simulink model "TestCase1_Modified"  (R2014a)
settings: Solver=FixedStepAuto  StartTime=0.0  StopTime=10.0  RelTol=1e-3
model workspace: external: MAT-File TestCase1.mat (data not in the file)
libraries: libAsserts x5
settings Model: Creator=Josef  LastModifiedBy=swami
settings DataIOCC: SaveFormat=Dataset
settings OptimizationCC: SimCompilerOptimization=off
settings DebuggingCC: MergeDetectMultiDrivingBlocksExec=error  SolverPrmCheckMsg=none  FrameProcessingCompatibilityMsg=error  AllowSymbolicDim=off
settings HardwareCC: ProdBitPerPointer=64  ProdLargestAtomicFloat=Float  ProdIntDivRoundTo=Zero  ProdEndianess=LittleEndian  ProdWordSize=64  ProdHWDeviceType=Intel->x86-64 (Windows64)
settings RTWCC: RTWCompilerOptimization=off
settings GRTTargetCC: GeneratePreprocessorConditionals=Use local settings
settings ConfigComp: CovMetricSettings=dw  CovHtmlReporting=on  CovSaveCumulativeToWorkspaceVar=on  CovSaveSingleToWorkspaceVar=on  CovExternalEMLEnable=off

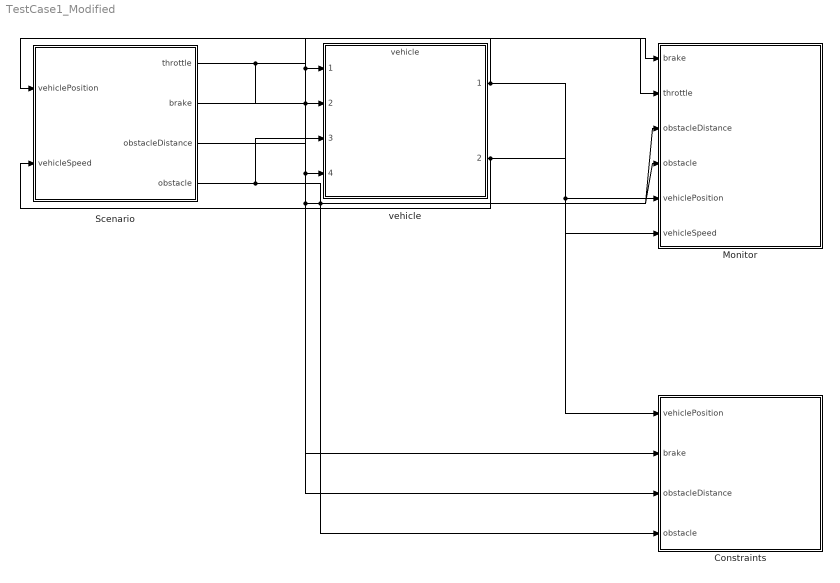
== system TestCase1_Modified ==
  Constraints : Subsystem
  Monitor : Subsystem
  Scenario : Subsystem
  vehicle : ModelReference  ModelNameDialog=vehicle  SimulationMode=Normal  ModelReferenceVersion=1.16  CopyOfModelName=vehicle  DefaultDataLogging=on
  wires:
  Scenario/1(throttle) -> vehicle/2, Monitor/2(throttle)
  Scenario/2(brake) -> vehicle/1, Monitor/1(brake), Constraints/2(brake)
  Scenario/4(obstacle) -> Monitor/4(obstacle), Constraints/4(obstacle), vehicle/3
  Scenario/3(obstacleDistance) -> Monitor/3(obstacleDistance), Constraints/3(obstacleDistance), vehicle/4
  vehicle/2 -> Scenario/2(vehicleSpeed), Monitor/6(vehicleSpeed)
  vehicle/1 -> Monitor/5(vehiclePosition), Constraints/1(vehiclePosition), Scenario/1(vehiclePosition)

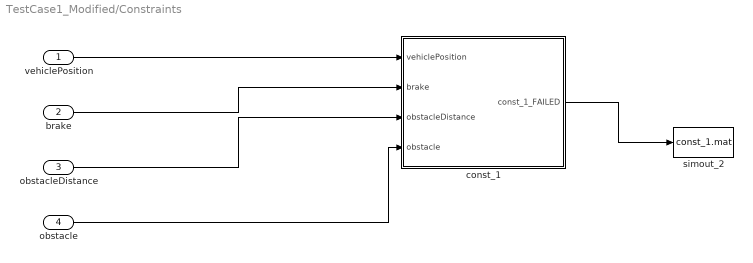
== system TestCase1_Modified/Constraints ==
  vehiclePosition : Inport
  brake : Inport  Port=2
  obstacleDistance : Inport  Port=3
  obstacle : Inport  Port=4
  const_1 : Subsystem
  simout_2 : ToFile  Filename=const_1.mat  MatrixName=const_1  SaveFormat=Timeseries
  wires:
  vehiclePosition/1 -> const_1/1(vehiclePosition)
  obstacleDistance/1 -> const_1/3(obstacleDistance)
  obstacle/1 -> const_1/4(obstacle)
  const_1/1(const_1_FAILED) -> simout_2/1
  brake/1 -> const_1/2(brake)

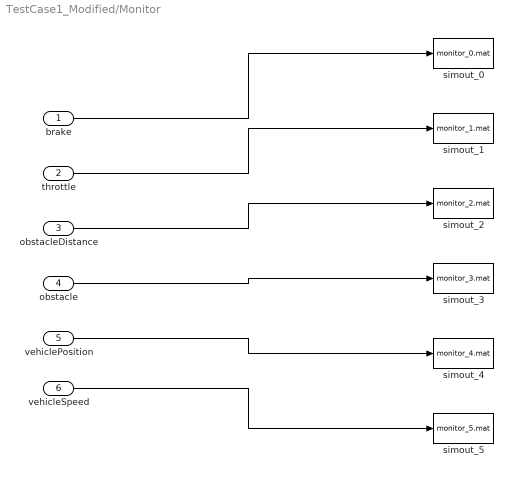
== system TestCase1_Modified/Monitor ==
  brake : Inport
  throttle : Inport  Port=2
  obstacleDistance : Inport  Port=3
  obstacle : Inport  Port=4
  vehiclePosition : Inport  Port=5
  vehicleSpeed : Inport  Port=6
  simout_0 : ToFile  Filename=monitor_0.mat  MatrixName=brake  SaveFormat=Timeseries
  simout_1 : ToFile  Filename=monitor_1.mat  MatrixName=throttle  SaveFormat=Timeseries
  simout_2 : ToFile  Filename=monitor_2.mat  MatrixName=obstacleDistance  SaveFormat=Timeseries
  simout_3 : ToFile  Filename=monitor_3.mat  MatrixName=obstacle  SaveFormat=Timeseries
  simout_4 : ToFile  Filename=monitor_4.mat  MatrixName=vehiclePosition  SaveFormat=Timeseries
  simout_5 : ToFile  Filename=monitor_5.mat  MatrixName=vehicleSpeed  SaveFormat=Timeseries
  wires:
  brake/1 -> simout_0/1
  throttle/1 -> simout_1/1
  obstacleDistance/1 -> simout_2/1
  obstacle/1 -> simout_3/1
  vehiclePosition/1 -> simout_4/1
  vehicleSpeed/1 -> simout_5/1

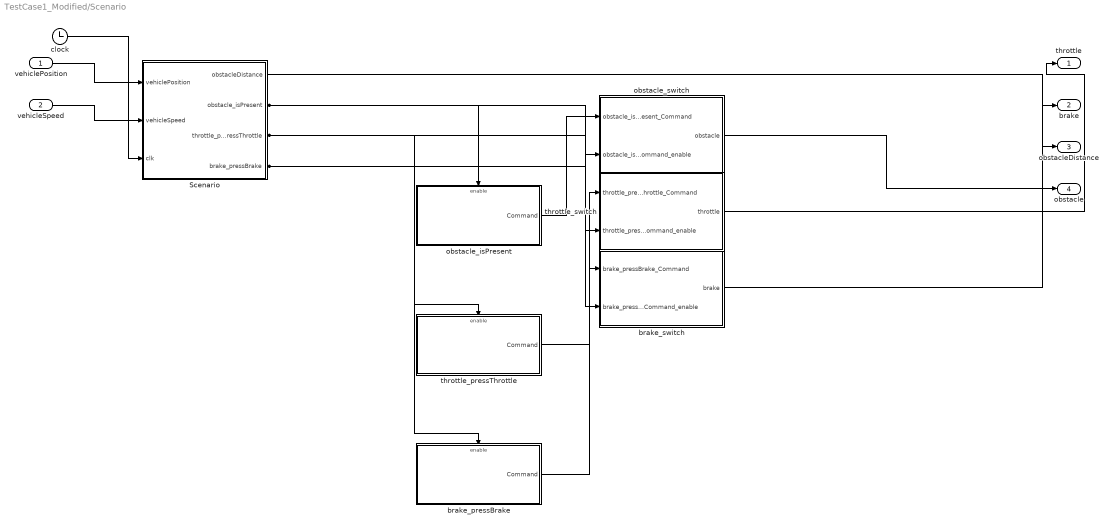
== system TestCase1_Modified/Scenario ==
  vehiclePosition : Inport
  vehicleSpeed : Inport  Port=2
  Scenario : Stateflow chart  TreatAsAtomicUnit=on
  brake_pressBrake : Subsystem
  brake_switch : Subsystem
  clock : Clock
  obstacle_isPresent : Subsystem
  obstacle_switch : Subsystem
  throttle_pressThrottle : Subsystem
  throttle_switch : Subsystem
  throttle : Outport
  brake : Outport  Port=2
  obstacleDistance : Outport  Port=3
  obstacle : Outport  Port=4
  wires:
  obstacle_switch/1(obstacle) -> obstacle/1
  throttle_switch/1(throttle) -> throttle/1
  brake_switch/1(brake) -> brake/1
  obstacle_isPresent/1(Command) -> obstacle_switch/1(obstacle_isPresent_Command)
  Scenario/2(obstacle_isPresent) -> obstacle_switch/2(obstacle_isPresent_Command_enable), obstacle_isPresent/Enable
  throttle_pressThrottle/1(Command) -> throttle_switch/1(throttle_pressThrottle_Command)
  Scenario/3(throttle_pressThrottle) -> throttle_switch/2(throttle_pressThrottle_Command_enable), throttle_pressThrottle/Enable
  brake_pressBrake/1(Command) -> brake_switch/1(brake_pressBrake_Command)
  Scenario/4(brake_pressBrake) -> brake_switch/2(brake_pressBrake_Command_enable), brake_pressBrake/Enable
  Scenario/1(obstacleDistance) -> obstacleDistance/1
  vehicleSpeed/1 -> Scenario/2(vehicleSpeed)
  vehiclePosition/1 -> Scenario/1(vehiclePosition)
  clock/1 -> Scenario/3(clk)

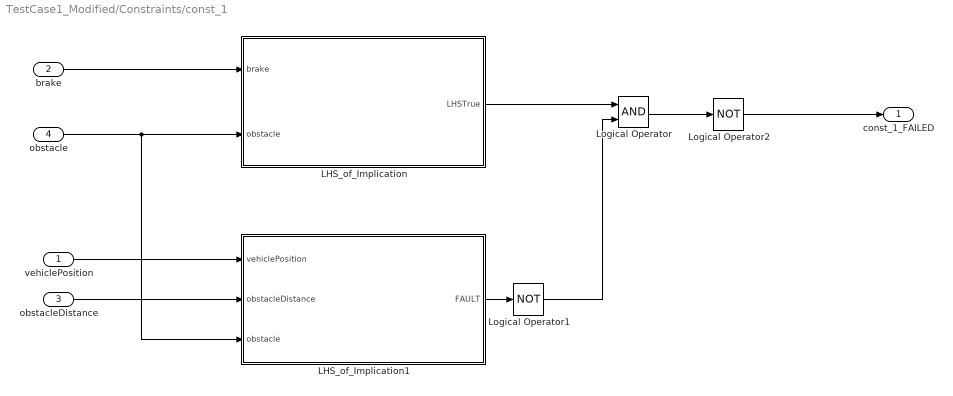
== system TestCase1_Modified/Constraints/const_1 ==
  vehiclePosition : Inport
  brake : Inport  Port=2
  obstacleDistance : Inport  Port=3
  obstacle : Inport  Port=4
  LHS_of_Implication : Subsystem
  LHS_of_Implication1 : Subsystem
  Logical Operator : Logic  AllPortsSameDT=off  OutDataTypeStr=boolean
  Logical Operator1 : Logic  Operator=NOT  AllPortsSameDT=off  OutDataTypeStr=boolean
  Logical Operator2 : Logic  Operator=NOT  AllPortsSameDT=off  OutDataTypeStr=boolean
  const_1_FAILED : Outport
  wires:
  brake/1 -> LHS_of_Implication/1(brake)
  obstacleDistance/1 -> LHS_of_Implication1/2(obstacleDistance)
  obstacle/1 -> LHS_of_Implication1/3(obstacle), LHS_of_Implication/2(obstacle)
  LHS_of_Implication1/1(FAULT) -> Logical Operator1/1
  LHS_of_Implication/1(LHSTrue) -> Logical Operator/1
  Logical Operator1/1 -> Logical Operator/2
  vehiclePosition/1 -> LHS_of_Implication1/1(vehiclePosition)
  Logical Operator/1 -> Logical Operator2/1
  Logical Operator2/1 -> const_1_FAILED/1

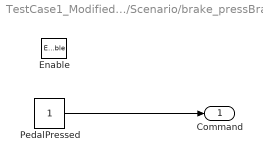
== system TestCase1_Modified/Scenario/brake_pressBrake ==
  Enable : EnablePort
  PedalPressed : Constant
  Command : Outport  OutputWhenDisabled=reset  InitialOutput=0
  wires:
  PedalPressed/1 -> Command/1

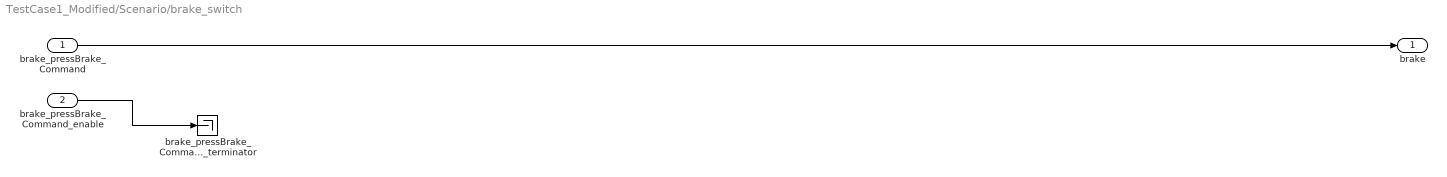
== system TestCase1_Modified/Scenario/brake_switch ==
  brake_pressBrake_Command : Inport
  brake_pressBrake_Command_enable : Inport  Port=2
  brake_pressBrake_Command_terminator : Terminator
  brake : Outport
  wires:
  brake_pressBrake_Command_enable/1 -> brake_pressBrake_Command_terminator/1
  brake_pressBrake_Command/1 -> brake/1

== system TestCase1_Modified/Scenario/obstacle_isPresent ==
  Enable : EnablePort
  PedalPressed : Constant
  Command : Outport  OutputWhenDisabled=reset  InitialOutput=0
  wires:
  PedalPressed/1 -> Command/1

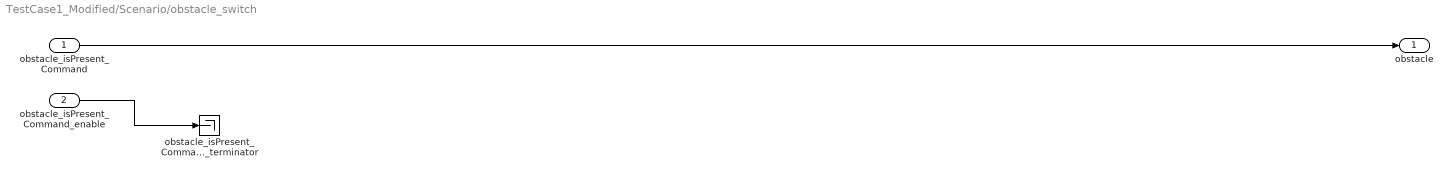
== system TestCase1_Modified/Scenario/obstacle_switch ==
  obstacle_isPresent_Command : Inport
  obstacle_isPresent_Command_enable : Inport  Port=2
  obstacle_isPresent_Command_terminator : Terminator
  obstacle : Outport
  wires:
  obstacle_isPresent_Command_enable/1 -> obstacle_isPresent_Command_terminator/1
  obstacle_isPresent_Command/1 -> obstacle/1

== system TestCase1_Modified/Scenario/throttle_pressThrottle ==
  Enable : EnablePort
  PedalPressed : Constant
  Command : Outport  OutputWhenDisabled=reset  InitialOutput=0
  wires:
  PedalPressed/1 -> Command/1

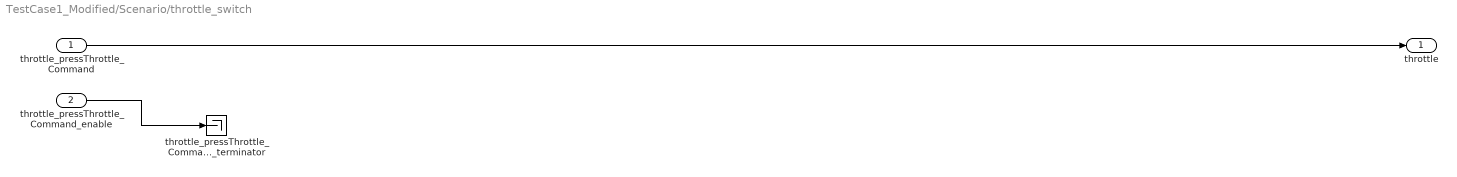
== system TestCase1_Modified/Scenario/throttle_switch ==
  throttle_pressThrottle_Command : Inport
  throttle_pressThrottle_Command_enable : Inport  Port=2
  throttle_pressThrottle_Command_terminator : Terminator
  throttle : Outport
  wires:
  throttle_pressThrottle_Command_enable/1 -> throttle_pressThrottle_Command_terminator/1
  throttle_pressThrottle_Command/1 -> throttle/1

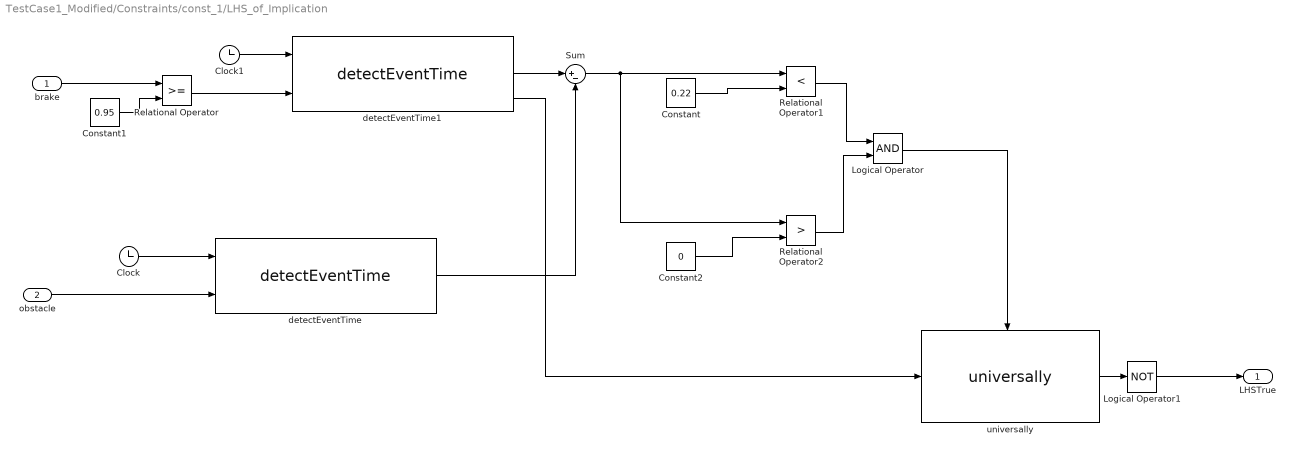
== system TestCase1_Modified/Constraints/const_1/LHS_of_Implication ==
  brake : Inport
  obstacle : Inport  Port=2
  Clock : Clock
  Clock1 : Clock
  Constant : Constant  Value=0.22
  Constant1 : Constant  Value=0.95
  Constant2 : Constant  Value=0
  Logical Operator : Logic  AllPortsSameDT=off  OutDataTypeStr=boolean
  Logical Operator1 : Logic  Operator=NOT  AllPortsSameDT=off  OutDataTypeStr=boolean
  Relational Operator : RelationalOperator  OutDataTypeStr=boolean
  Relational Operator1 : RelationalOperator  Operator=<  OutDataTypeStr=boolean
  Relational Operator2 : RelationalOperator  Operator=>  OutDataTypeStr=boolean
  Sum : Sum  Inputs=|+-
  detectEventTime : libAsserts/detectEventTime
  detectEventTime1 : libAsserts/detectEventTime
  universally : libAsserts/universally
  LHSTrue : Outport
  wires:
  detectEventTime1/2 -> Sum/1
  obstacle/1 -> detectEventTime/2
  universally/1 -> Logical Operator1/1
  Constant2/1 -> Relational Operator2/2
  Logical Operator1/1 -> LHSTrue/1
  Logical Operator/1 -> universally/Enable
  detectEventTime1/3 -> universally/1
  Sum/1 -> Relational Operator2/1, Relational Operator1/1
  Constant/1 -> Relational Operator1/2
  Relational Operator/1 -> detectEventTime1/2
  Clock1/1 -> detectEventTime1/1
  brake/1 -> Relational Operator/1
  Relational Operator1/1 -> Logical Operator/1
  detectEventTime/2 -> Sum/2
  Relational Operator2/1 -> Logical Operator/2
  Constant1/1 -> Relational Operator/2
  Clock/1 -> detectEventTime/1

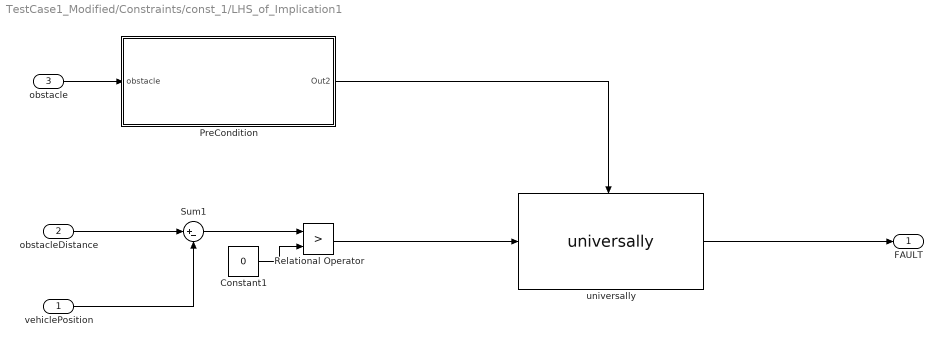
== system TestCase1_Modified/Constraints/const_1/LHS_of_Implication1 ==
  vehiclePosition : Inport
  obstacleDistance : Inport  Port=2
  obstacle : Inport  Port=3
  Constant1 : Constant  Value=0
  PreCondition : Subsystem
  Relational Operator : RelationalOperator  Operator=>  OutDataTypeStr=boolean
  Sum1 : Sum  Inputs=|+-
  universally : libAsserts/universally
  FAULT : Outport
  wires:
  Constant1/1 -> Relational Operator/2
  universally/1 -> FAULT/1
  obstacle/1 -> PreCondition/1(obstacle)
  obstacleDistance/1 -> Sum1/1
  vehiclePosition/1 -> Sum1/2
  Sum1/1 -> Relational Operator/1
  Relational Operator/1 -> universally/1
  PreCondition/1(Out2) -> universally/Enable

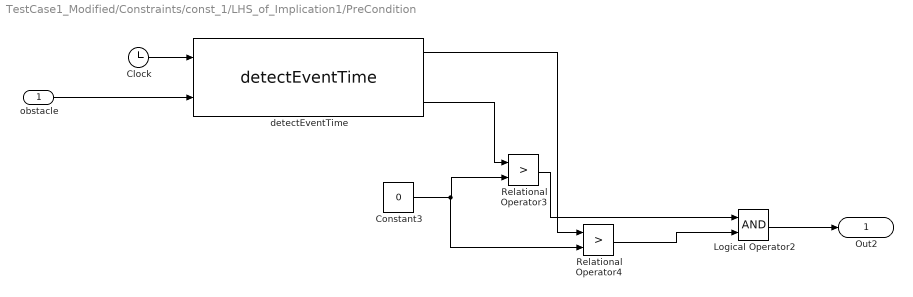
== system TestCase1_Modified/Constraints/const_1/LHS_of_Implication1/PreCondition ==
  obstacle : Inport
  Clock : Clock
  Constant3 : Constant  Value=0
  Logical Operator2 : Logic  AllPortsSameDT=off  OutDataTypeStr=boolean
  Relational Operator3 : RelationalOperator  Operator=>  OutDataTypeStr=boolean
  Relational Operator4 : RelationalOperator  Operator=>  OutDataTypeStr=boolean
  detectEventTime : libAsserts/detectEventTime
  Out2 : Outport
  wires:
  Clock/1 -> detectEventTime/1
  obstacle/1 -> detectEventTime/2
  Relational Operator3/1 -> Logical Operator2/1
  detectEventTime/1 -> Relational Operator4/1
  detectEventTime/3 -> Relational Operator3/1
  Constant3/1 -> Relational Operator4/2, Relational Operator3/2
  Logical Operator2/1 -> Out2/1
  Relational Operator4/1 -> Logical Operator2/2

== stateflow chart TestCase1_Modified/Scenario/Scenario ==
  state Act_Driver [parallel]
    settings: executionOrder=1
    state Act_Driver_Step1
      state Act_Driver_Step1_1
        entry: throttle_pressThrottle = 1;
      state Act_Driver_Step1_2
        entry: throttle_pressThrottle = 0;
      (default) -> Act_Driver_Step1_1
      Act_Driver_Step1_1 -> Act_Driver_Step1_2 : [vehicleSpeed >= 50]
    state Act_Driver_Step2
    state Act_Driver_Step3
      entry: Act_Driver_Step3_stpClk = clk;
    state Act_Driver_Step4
      entry: brake_pressBrake = 1;
    (default) -> Act_Driver_Step1
    Act_Driver_Step1 -> Act_Driver_Step2
    Act_Driver_Step2 -> Act_Driver_Step3 : [obstacle_isPresent]
    Act_Driver_Step3 -> Act_Driver_Step4 : [clk - Act_Driver_Step3_stpClk > 0.21]
  state Act_Obstacle [parallel]
    settings: executionOrder=2
    state Act_Obstacle_Step1
      entry: obstacle_isPresent = 0;
      entry: Act_Obstacle_Step1_stpClk = clk;
    state Act_Obstacle_Step2
      entry: obstacle_isPresent = 1;
      entry: obstacleDistance = 50 + vehiclePosition;
    (default) -> Act_Obstacle_Step1
    Act_Obstacle_Step1 -> Act_Obstacle_Step2 : [clk - Act_Obstacle_Step1_stpClk > 5]
  data: vehiclePosition input; vehicleSpeed input; clk input; obstacleDistance output; obstacle_isPresent output; throttle_pressThrottle output; brake_pressBrake output; Act_Driver_Step3_stpClk local; Act_Obstacle_Step1_stpClk local
